simulink model "ControlPlantaCompleta"  (R2020a)
settings: Solver=VariableStepAuto  StartTime=0.0  StopTime=10.0  RelTol=1e-3
libraries: simulink x1
settings Model: Creator=MI PC  LastModifiedBy=aldajo92

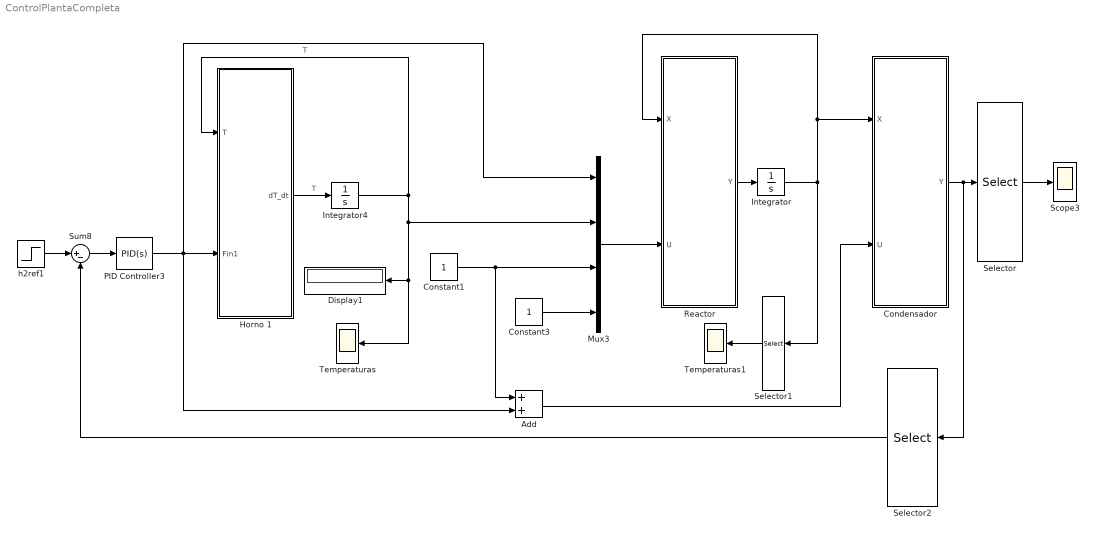
== system ControlPlantaCompleta ==
  Add : Sum
  Condensador : MATLAB Function  TreatAsAtomicUnit=on
  Constant1 : Constant
  Constant3 : Constant
  Display1 : Display
  Horno 1 : MATLAB Function  TreatAsAtomicUnit=on
  Integrator : Integrator  InitialCondition=[1;1;1;1;1;1;7]
  Integrator4 : Integrator
  Mux3 : Mux
  PID Controller3 : simulink/Continuous/PID Controller  Controller=PID  Form=Parallel  TimeDomain=Continuous-time  UseExternalTs=off  SampleTime=1  IntegratorMethod=Forward Euler  FilterMethod=Forward Euler  ControllerParametersSource=internal  P=5  I=0  D=-1  UseFilter=on  N=100  TunerSelectOption=Transfer Function Based (PID Tuner App)  InitialConditionSource=internal  InitialConditionForIntegrator=0  InitialConditionForFilter=0  DifferentiatorICPrevScaledInput=0  ExternalReset=none  TrackingMode=off  Kt=1  LimitOutput=off  UpperSaturationLimit=inf  LowerSaturationLimit=-inf  LinearizeAsGain=off  AntiWindupMode=none  Kb=1  POutMin=[]  POutMax=[]  IOutMin=[]  IOutMax=[]  DOutMin=[]  DOutMax=[]  NOutMin=[]  NOutMax=[]  SumOutMin=[]  SumOutMax=[]  SaturationOutMin=[]  SaturationOutMax=[]  PParamMin=[]  PParamMax=[]  IParamMin=[]  IParamMax=[]  DParamMin=[]  DParamMax=[]  NParamMin=[]  NParamMax=[]  KbParamMin=[]  KbParamMax=[]  KtParamMin=[]  KtParamMax=[]  KbOutMin=[]  KbOutMax=[]  KtOutMin=[]  KtOutMax=[]  IntegratorOutMin=[]  IntegratorOutMax=[]  FilterOutMin=[]  FilterOutMax=[]  SumI1OutMin=[]  SumI1OutMax=[]  SumI2OutMin=[]  SumI2OutMax=[]  SumI3OutMin=[]  SumI3OutMax=[]  SumI4OutMin=[]  SumI4OutMax=[]  SumDOutMin=[]  SumDOutMax=[]  DifferentiatorOutMin=[]  DifferentiatorOutMax=[]  FilterDiffOutCoefMin=[]  FilterDiffOutCoefMax=[]  ReciprocalOutMin=[]  ReciprocalOutMax=[]  SumDenOutMin=[]  SumDenOutMax=[]  SumNumOutMin=[]  SumNumOutMax=[]  DivideOutMin=[]  DivideOutMax=[]  UdiffTsProdOutMin=[]  UdiffTsProdOutMax=[]  NTsProdOutMin=[]  NTsProdOutMax=[]  UintegralTsProdOutMin=[]  UintegralTsProdOutMax=[]  UngainTsProdOutMin=[]  UngainTsProdOutMax=[]  IntegratorContinuousStateAttributes=''  IntegratorStateMustResolveToSignalObject=off  IntegratorRTWStateStorageClass=Auto  FilterContinuousStateAttributes=''  FilterStateMustResolveToSignalObject=off  FilterRTWStateStorageClass=Auto  ParallelPVariant=InternalParameters  IdealPVariant=Disabled  IVariant=InternalParameters  DVariant=InternalParameters  IntegratorVariant=Continuous  SatVariant=Disabled  AWVariant=Passthrough  PCopyVariant=Disabled  TRVariant=Disabled  FdbkBlocksVariant=Forward  IdealPFdbkVariant=Disabled  SatFdbkVariant=Disabled  DerivativeFilterVariant=ContFilter  NVariant=InternalParameters  NCopyVariant=Disabled  FilterICVariant=InternalICsFilter  IntegratorICVariant=InternalICs  ExternalResetVariant=Disabled  TRSumVariant=Passthrough  SumFdbkVariant=Disabled  SumVariant=Sum_PID  TsampFilterVariant=InternalTs  TsampNgainVariant=Passthrough  TsampIntegralVariant=Passthrough
  Reactor : MATLAB Function  TreatAsAtomicUnit=on
  Scope3 : Scope
  Selector : Selector  InputPortWidth=7  IndexOptions=Index vector (dialog)  Indices=[1 3 4]  OutputSizes=1
  Selector1 : Selector  InputPortWidth=7  IndexOptions=Index vector (dialog)  Indices=[1 3 4]  OutputSizes=1
  Selector2 : Selector  InputPortWidth=7  IndexOptions=Index vector (dialog)  Indices=[3]  OutputSizes=1
  Sum8 : Sum  Inputs=|+-
  Temperaturas : Scope
  Temperaturas1 : Scope
  h2ref1 : Step  Time=5  Before=200  After=300  SampleTime=0
  wires:
  Integrator4/1 -> Mux3/2, Temperaturas/1, Display1/1, Horno 1/1(T)  "T"
  Horno 1/1(dT_dt) -> Integrator4/1  "T"
  Integrator/1 -> Selector1/1, Reactor/1(X), Condensador/1(X)
  Reactor/1(Y) -> Integrator/1
  Mux3/1 -> Reactor/2(U)
  Constant3/1 -> Mux3/4
  Add/1 -> Condensador/2(U)
  PID Controller3/1 -> Add/2, Mux3/1, Horno 1/2(Fin1)
  Constant1/1 -> Add/1, Mux3/3
  Condensador/1(Y) -> Selector2/1, Selector/1
  Selector/1 -> Scope3/1
  Selector1/1 -> Temperaturas1/1
  Sum8/1 -> PID Controller3/1
  Selector2/1 -> Sum8/2
  h2ref1/1 -> Sum8/1

== matlab function ControlPlantaCompleta/Reactor ==
  data: X input; Y output; U input
function Y = Reactor(X, U)
    %% Mapeo de variables
    Ca = X(1);
    Cb = X(2);
    Cc = X(3);
    Cd = X(4);
    Ce = X(5);
    Cf = X(6);
    T  = X(7);
    
    Fin1  = U(1);
    Fin2  = U(2);
    T_Ain = U(3);
    T_Bin = U(4);
    
    %% parametros reactor
    V = 20;

    Tin = 298;
    Top = 298;
    UA = 34;

    Fout = Fin1 + Fin2;
    ci0 = [10;10;0;0;0;0];
    
    R = 0.082;
    Ta = 298;
    Tref = Ta;
    P_A = 1;
    P_B = 1;
    
    r_1 = 1.00*(10^6)*exp(-22500/(R*T))*Ca*Cb;
    r_2 = 6.00*(10^5)*exp(-22500/(R*T))*Cb*Cc;
    r_3 = 7.80*(10^6)*exp(-25000/(R*T))*Ca*Cd;
    r_4 = 1.80*(10^8)*exp(-20000/(R*T))*(Cb^2)*Ce;
    
    r_i = [r_1;r_2;r_3;r_4];
    delta_H_r_i = [-114;0;0;0];
    
    r_gen_i = [
        0;
        0;
        r_1 + r_3 + r_4;
        r_2;
        0;
        r_4
        ];
    
    r_con_i = [
        r_1 + (r_3/2);
        r_1 + r_2 + (2*r_4);
        r_2;
        (r_3/2);
        r_4;
        0
        ];
    
    CpA = 0.08167;      % [KJ/mol K] Calor especifico monoxido de carbono
    CpB = 0.04284;      % [KJ/mol K] Calor especifico hidrogeno
    CpC = 0.12841;      % [KJ/mol K] Calor especifico dioxido de carbono
    CpD = 0.25729;      % [KJ/mol K] Calor especifico metanol
    CpE = 0.15723;      % [KJ/mol K] Calor especifico dioxido de carbono
    CpF = 0.06431;      % [KJ/mol K] Calor especifico agua
    
    wa = 0.07812;
    wb = 0.02805;
    wc = 0.13422;
    wd = 0.10616;
    we = 0.09214;
    wf = 0.04208;
    
    ro_A = P_A*wa/(R*T_Ain);
    ro_B = P_B*wb/(R*T_Bin);
    
    Ha_in = CpA * (T_Ain - T);
    Hb_in = CpB * (T_Bin - T);
    
    Ha = CpA * (T - Ta);
    Hb = CpB * (T - Ta);
    Hc = CpC * (T - Ta);
    Hd = CpD * (T - Ta);
    He = CpE * (T - Ta);
    Hf = CpF * (T - Ta);
    
    dCa_dt = (Fin1*ci0(1) - Fout*Ca)/V + r_gen_i(1) - r_con_i(1);
    dCb_dt = (Fin2*ci0(2) - Fout*Cb)/V + r_gen_i(2) - r_con_i(2);
    dCc_dt = (Fin1*ci0(3) - Fout*Cc)/V + r_gen_i(3) - r_con_i(3);
    dCd_dt = (Fin1*ci0(4) - Fout*Cd)/V + r_gen_i(4) - r_con_i(4);
    dCe_dt = (Fin1*ci0(5) - Fout*Ce)/V + r_gen_i(5) - r_con_i(5);
    dCf_dt = (Fin1*ci0(6) - Fout*Cf)/V + r_gen_i(6) - r_con_i(6);
    
    Q = 34*(300-Tref);
    sumDeltaHrs = V*(r_i'*delta_H_r_i);
    
    sumCiHi = Ca*Ha + Cb*Hb + Cc*Hc + Cd*Hd + Ce*He + Cf*Hf;
    dT_dt_num = (Fin1*ro_A*Ha) + (Fin2*ro_B*Hb) - (Fout*sumCiHi) + Q - sumDeltaHrs;
    dT_dt_den = (ro_A*CpA + ro_B*CpB)*V;
    
    dT_dt = dT_dt_num/dT_dt_den;
    
    Y = [dCa_dt; dCb_dt; dCc_dt; dCd_dt; dCe_dt; dCf_dt; dT_dt]
end

== matlab function ControlPlantaCompleta/Horno 1 ==
  data: T input; dT_dt output; Fin1 input
function dT_dt = horno(T, Fin1)
    %% parametros planta horno
    V = 10;
    Tin = 298;
    Top = 400;
    rho_a = 1;
    UA = 35;
    rho_a = 1;
    Cp = 1;
    
    dT_dt = (Fin1*(Tin - T)/V) - (UA*(Top - T)/(rho_a*V*Cp));

end

== matlab function ControlPlantaCompleta/Condensador ==
  data: X input; Y output; U input
function Y = Condensador(X, U)
    Ca = X(1);
    Cb = X(2);
    Cc = X(3);
    Cd = X(4);
    Ce = X(5);
    Cf = X(6);
    T  = X(7);
    
    Y = [Ca*U; 0; Cc*U; Cd*U; 0; 0; 270];
end
